simulink model "CosimSpeedSimulationHw"  (R2013b)
settings: Solver=FixedStepDiscrete  SolverMode=SingleTasking  StartTime=0.0  StopTime=inf  FixedStep=0.1  RelTol=1e-3
undefined symbols (not defined in the file or in its folder): A, N
libraries: xbsIndex_r4 x1, JTAGRuntimeCosim_r4 x1
settings Model: Creator=laca  LastModifiedBy=laca

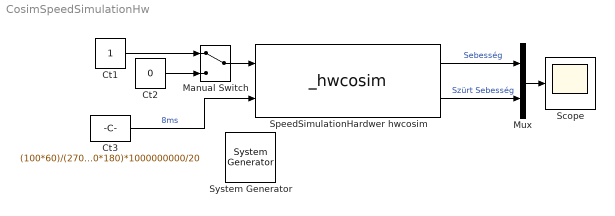
== system CosimSpeedSimulationHw ==
  " System Generator" : xbsIndex_r4/ System Generator  Tag=genX  xilinxfamily=spartan3e  part=xc3s500e  speed=-4  package=pq208  synthesis_tool=XST  clock_wrapper=Clock Enables  directory=./netlist  proj_type=Project Navigator  Synth_file=XST Defaults  Impl_file=ISE Defaults  testbench=off  simulink_period=1  sysclk_period=20  dcm_input_clock_period=10  incr_netlist=off  trim_vbits=Everywhere in SubSystem  dbl_ovrd=According to Block Masks  core_generation=According to Block Masks  run_coregen=off  deprecated_control=off  eval_field=0  block_type=sysgen
  Ct1 : Constant
  Ct2 : Constant  Value=0
  Ct3 : Constant  Value=(100*60)/(2700*180)*1000000000/20
  Manual Switch : ManualSwitch
  Mux : Mux  Inputs=2
  Scope : Scope
      settings: TickLabels=on  ShowLegends=on  YMin=-80  YMax=0
  SpeedSimulationHardwer hwcosim : JTAGRuntimeCosim_r4/_hwcosim  clkSrc=Free Running  hasCombinationalPath=off  bitfileName=C:\Diak\gl\SPARTAN3E500K_slave\SystemGenrator\SebessegEsPozicio\netlist\speedsimulationhardwer_cw.bit  skipConfig=off  cable=Auto Detect  speed=N/A  cablePort=N/A  cableLocation=Local  shareCable=off  enable_codebug=on  design_xtable=|  engineDll=JTAGCosimEngine.dll  cableWaitTime=10  bscanPos=1  IRLengths=[6,8]  useWaitBox=1  hasBufgmux=on  Scheme=Cosim  useCmdProc=1  hasProc=0  useImpact=0  printLogFile=0  block_type=jtagcosim
      | {
      |   'clkWrapper' => 'speedsimulationhardwer_cw',
      |   'clocksGcd' => undef,
      |   'device' => 'xc3s500e-4pq208',
      |   'ports' => {
      |     'cseredir' => {
      |       'bd_port_index' => 0,
      |       'direction' => 'in',
      |       'icon_text' => 'CsereDir',
      |       'period' => 1,
      |       'sim_pause_trigger' => false,
      |       'type' => 'Bool',
      |       'width' => 1,
      |     },
      |     'sebess_g' => {
      |       'bd_port_index' => 0,
      |       'direction' => 'out',
      |       'icon_text' => 'Sebesség',
      |       'period' => 1,
      |       'sim_pause_trigger' => false,
      |       'type' => 'Fix_16_0',
      |       'width' => 16,
      |     },
      |     'sz_rtsebess_g' => {
      |       'bd_port_index' => 1,
      |       'direction' => 'out',
      |       'icon_text' => 'SzürtSebesség',
      |       'period' => 1,
      |       'sim_pause_trigger' => false,
      |       'type' => 'Fix_16_0',
      |       'width' => 16,
      |     },
      |     'tsval' => {
      |       'bd_port_index' => 1,
      |       'direction' => 'in',
      |       'icon_text' => 'TSval',
      |       'period' => 1,
      |       'sim_pause_trigger' => false,
      |       'type' => 'UFix_32_0',
      |       'width' => 32,
      |     },
      |   },
      |   'shared_memories' => {},
      | }
  wires:
  Ct1/1 -> Manual Switch/1
  Ct2/1 -> Manual Switch/2
  SpeedSimulationHardwer hwcosim/1 -> Mux/1  "Sebesség"
  SpeedSimulationHardwer hwcosim/2 -> Mux/2  "Szürt Sebesség"
  Mux/1 -> Scope/1
  Manual Switch/1 -> SpeedSimulationHardwer hwcosim/1
  Ct3/1 -> SpeedSimulationHardwer hwcosim/2  "8ms"
